simulink model "scheme1"  (R2024a)
settings: Solver=FixedStepAuto  StartTime=0.0  StopTime=10  FixedStep=10e-4  RelTol=1e-6
undefined symbols (not defined in the file or in its folder): a, b, c, k, T, w, y1
settings Model: Creator=alexivanov  LastModifiedBy=alexivanov

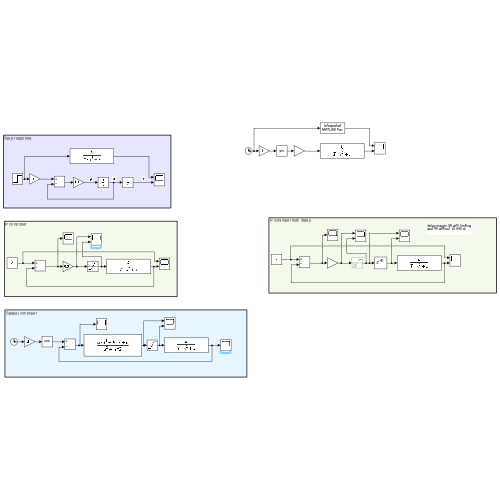
[thumbnail: Simulink's stored preview of the top-level diagram]
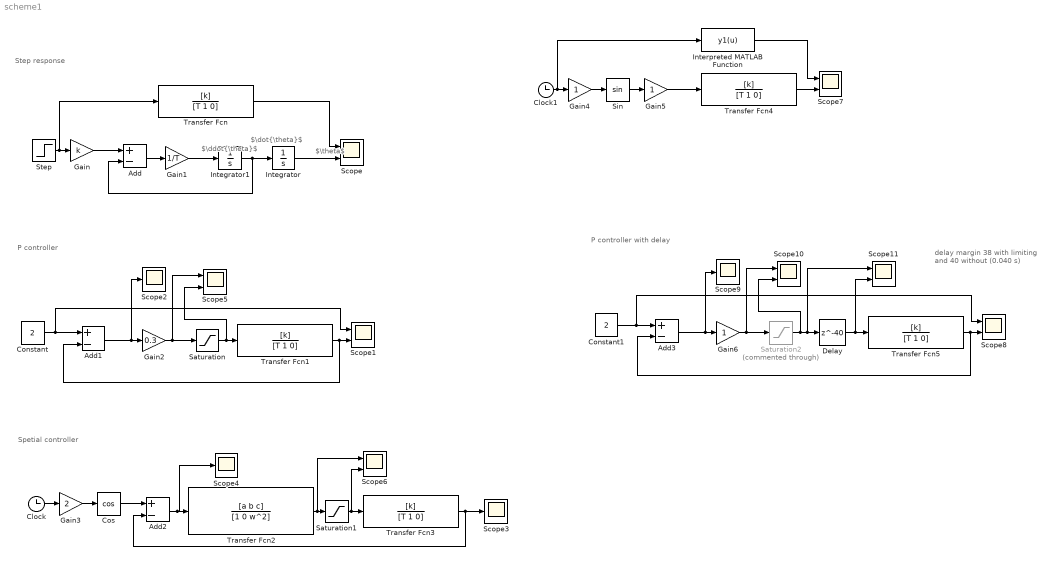
== system scheme1 ==
  note: delay margin 38 with limiting
      | and 40 without  (0.040 s)
  note: Spetial controller
  note: P controller
  note: Step response
  note: $\theta$
  note: $\dot{\theta}$
  note: $\ddot{\theta}$
  note: P controller with delay
  Add{,1..3} (4 alike) : Sum  Inputs=+-
  Clock : Clock
  Clock1 : Clock
  Constant : Constant  Value=2
  Constant1 : Constant  Value=2
  Cos : Trigonometry  Operator=cos
  Delay : Delay  DelayLength=40
  Gain : Gain  Gain=k
  Gain1 : Gain  Gain=1/T
  Gain2 : Gain  Gain=0.3
  Gain3 : Gain  Gain=2
  Gain4 : Gain
  Gain5 : Gain
  Gain6 : Gain
  Integrator : Integrator
  Integrator1 : Integrator
  Interpreted MATLAB Function : MATLABFcn  MATLABFcn=y1(u)
  Saturation : Saturate  UpperLimit=1  LowerLimit=-1
  Saturation1 : Saturate  UpperLimit=1  LowerLimit=-1
  Saturation2 : Saturate  Commented=through  UpperLimit=1  LowerLimit=-1
  Scope{,1,5..8,10..11} (8 alike) : Scope  NumInputPorts=2
  Scope{2..4,9} (4 alike) : Scope
  Sin : Trigonometry
  Step : Step  Time=0  SampleTime=0
  Transfer Fcn{,1,3..5} (5 alike) : TransferFcn  Numerator=[k]  Denominator=[T 1 0]
  Transfer Fcn2 : TransferFcn  Numerator=[a b c]  Denominator=[1 0 w^2]
  wires:
  Integrator/1 -> Scope/2
  Integrator1/1 -> Add/2, Integrator/1
  Step/1 -> Transfer Fcn/1, Gain/1
  Gain/1 -> Add/1
  Add/1 -> Gain1/1
  Gain1/1 -> Integrator1/1
  Transfer Fcn/1 -> Scope/1
  Gain2/1 -> Saturation/1, Scope5/1
  Constant/1 -> Scope1/1, Add1/1
  Transfer Fcn1/1 -> Add1/2, Scope1/2
  Add1/1 -> Scope2/1, Gain2/1
  Clock/1 -> Gain3/1
  Gain3/1 -> Cos/1
  Cos/1 -> Add2/1
  Add2/1 -> Scope4/1, Transfer Fcn2/1
  Transfer Fcn3/1 -> Scope3/1, Add2/2
  Saturation/1 -> Scope5/2, Transfer Fcn1/1
  Transfer Fcn2/1 -> Scope6/1, Saturation1/1
  Saturation1/1 -> Scope6/2, Transfer Fcn3/1
  Clock1/1 -> Interpreted MATLAB Function/1, Gain4/1
  Gain4/1 -> Sin/1
  Sin/1 -> Gain5/1
  Gain5/1 -> Transfer Fcn4/1
  Transfer Fcn4/1 -> Scope7/2
  Interpreted MATLAB Function/1 -> Scope7/1
  Constant1/1 -> Scope8/1, Add3/1
  Transfer Fcn5/1 -> Add3/2, Scope8/2
  Add3/1 -> Scope9/1, Gain6/1
  Saturation2/1 -> Scope10/2, Scope11/1, Delay/1
  Gain6/1 -> Saturation2/1, Scope10/1
  Delay/1 -> Scope11/2, Transfer Fcn5/1
